simulink library "rotationAboutY"  (R2020a)
settings: Solver=VariableStepAuto  StartTime=0.0  StopTime=10.0  RelTol=1e-3
libraries: sharedutil x1
settings Model: Creator=Ayaz  LastModifiedBy=Ayaz

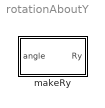
== system rotationAboutY ==
  makeRy : Subsystem

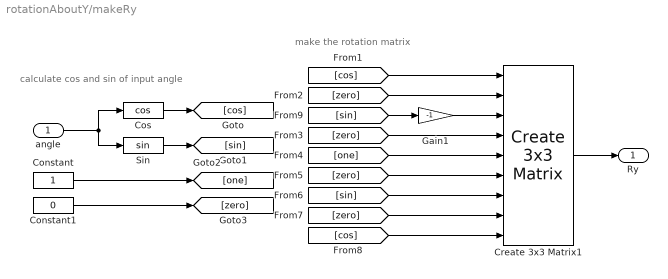
== system rotationAboutY/makeRy ==
  note: make the rotation matrix
  note: calculate cos and sin of input angle
  angle : Inport
  Constant : Constant  VectorParams1D=off
  Constant1 : Constant  Value=0  VectorParams1D=off
  Cos : Trigonometry  Operator=cos
  Create 3x3 Matrix1 : sharedutil/Create 3x3 Matrix  aMode=aMode
      settings: SourceProductBaseCode=AE,PW,MT,VE,VP
  Gain1 : Gain  Gain=-1
  Sin : Trigonometry
  Ry : Outport
  wires:
  [cos] -> Create 3x3 Matrix1/1
  [zero] -> Create 3x3 Matrix1/2
  [zero] -> Create 3x3 Matrix1/4
  [one] -> Create 3x3 Matrix1/5
  [zero] -> Create 3x3 Matrix1/6
  [sin] -> Create 3x3 Matrix1/7
  [zero] -> Create 3x3 Matrix1/8
  [cos] -> Create 3x3 Matrix1/9
  Create 3x3 Matrix1/1 -> Ry/1
  Gain1/1 -> Create 3x3 Matrix1/3
  Sin/1 -> [sin]
  Constant1/1 -> [zero]
  angle/1 -> Sin/1, Cos/1
  Constant/1 -> [one]
  Cos/1 -> [cos]
  [sin] -> Gain1/1
